simulink model "fscsim5"  (Simulink 3.00)
settings: Solver=ode45  SolverMode=SingleTasking  StartTime=0.0  StopTime=20e-3  MaxStep=Ts/10  RelTol=1e-3  AbsTol=1e-6
values from neighbouring files (symbols this model uses):
  sysd_P = c2d(ssbal(sys_P),Ts/10)    [seekdemo.m]
  Ts = PlantDataSeek.Ts    [seekdemo.m]
libraries: cstextras x2
settings Model: RTWOptions="-aEnforceIntegerDowncast=1 -aExtMode=0 -aExtModeTesting=0 -aFoldNonRolledExpr=1 -aForceParamTrailComments=0 -aGenerateComments=1 -aGenerateReport=0 -aIgnoreCustomStorageClasses=0 -aIncDataTypeInIds=0 -aIncHierarchyInIds=0 -aInlineInvariantSignals=1 -aInlinedPrmAccess=\"Literals\" -aLocalBlockOutputs=1 -aLogVarNameModifier=\"rt_\" -aMaxRTWIdLen=31 -aPrefixModelToSubsysFcnNames=1 -aRTWVerbose=1 -aRollThreshold=5 -aShowEliminatedStatements=0"  ExtModeTrigMode=normal  ExtModeArmWhenConnect=on  LastModifiedBy=takeyori

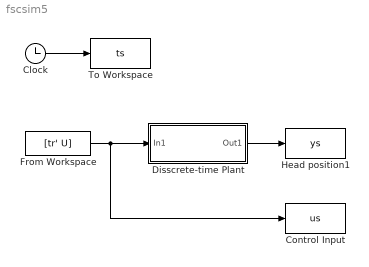
== system fscsim5 ==
  Clock : Clock
      settings: DisplayTime=off  Decimation=10
  Control Input : ToWorkspace  VariableName=us  SampleTime=Ts/10  SaveFormat=Matrix
  Disscrete-time Plant : Subsystem  mask(LTI Block){sys=sysd_P, IC=[0]}
      mask prompts: sys "LTI system variable"; IC "Initial states   (state-space only)"
      mask help:
      | The LTI System block accepts both continuous and discrete LTI objects as defined in the Control System Toolbox. Transfer function, state-space, and zero-pole-gain formats are all supported in this block.
      |
      | Note: For multi-input systems, the input delays must be either all positive or all zero.
      |
      | Note: Initial states are only meaningful for state-space systems.
      mask init:
      | sysname='???';
      | if ~exist('A'),
      | A=[];B=[];C=[];D=1;Xo=0;
      | end,
      | [A,B,C,D,Xo,Tdi,Tdo,Ts,sysname]=ltimask('AssignData',gcb,sys,IC);
      | ltimask( 'UpdateDiagram',gcb,sys,Tdi,Tdo);
      mask Help:
      | The LTI System block accepts any of the three standard LTI objects described in the Control System Toolbox: transfer function, zero/pole/gain, or state space. Internally, the object will be converted to its state space equivalent for evaluation.
      | <p>
      | In the editable text box labeled <b>LTI System Variable</b>, enter the variable name of an LTI object.
      | <p>
      | In the editable text box labeled <b>Initial States</b> enter the initial state vector for state-space systems only.
      |  <p>
      | <I>NOTE:</I> Initial states are only valid for state-space systems. The simulation will not run if non-zero initial states are given for transfer function or zero/pole/gain LTI objects
      | <p>
      | <I>NOTE:</b> For multi-input systems, the input delays (stored within the LTI object field: Td) must be either all positive or all zero. The simulation will not run if there is a mix of positive and zero input delays.
      | <p>
      | See also TF, ZPK, SS.
      mask CallbackString: ltimask('MaskLTICallback',gcb);|ltimask('MaskICCallback',gcb);
      mask Display: disp(sysname)
  From Workspace : FromWorkspace  VariableName=[tr' U]  SampleTime=Ts  Interpolate=off  HoldFinalValue=off
  Head position1 : ToWorkspace  VariableName=ys  SampleTime=Ts/10  SaveFormat=Matrix
  To Workspace : ToWorkspace  VariableName=ts  SampleTime=Ts/10  SaveFormat=Matrix
  wires:
  Clock/1 -> To Workspace/1
  Disscrete-time Plant/1(Out1) -> Head position1/1
  From Workspace/1 -> Disscrete-time Plant/1(In1), Control Input/1

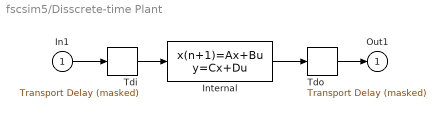
== system fscsim5/Disscrete-time Plant ==
  In1 : Inport  Port=1  PortWidth=-1  SampleTime=-1  DataType=auto
      settings: SignalType=auto
  Internal : DiscreteStateSpace  A=A  B=B  C=C  D=D  X0=Xo  SampleTime=Ts
  Tdi : cstextras/Transport Delay (masked)  Tag=InputDelayBlock  Td=Tdi  u0=0  bufsize=1024
  Tdo : cstextras/Transport Delay (masked)  Tag=OutputDelayBlock  Td=Tdo  u0=0  bufsize=1024
  Out1 : Outport  Port=1  InitialOutput=0
  wires:
  Tdo/1 -> Out1/1
  Internal/1 -> Tdo/1
  Tdi/1 -> Internal/1
  In1/1 -> Tdi/1
